simulink model "szalwach_mroz_perlinski"  (R2015a)
settings: Solver=ode45  StartTime=0.0  StopTime=200  RelTol=1e-3
settings Model: Creator=bszal  LastModifiedBy=bszal

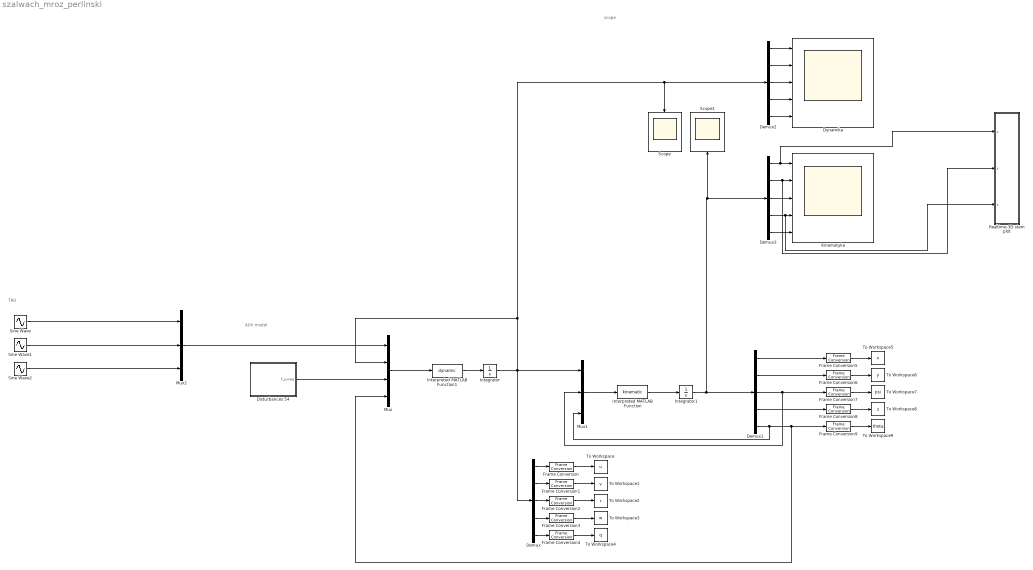
== system szalwach_mroz_perlinski ==
  note: scope
  note: TAU
  note: AUV model
  Demux{,1..3} (4 alike) : Demux  Outputs=5
  Disturbances 54 : Subsystem
  "Dynamika " : Scope  NumInputPorts=5
      settings: YMin=-5~-5~-5~-5~-5  YMax=5~5~5~5~5
  Frame Conversion{,1..9} (10 alike) : FrameConversion  OutFrame=Sample-based
  Integrator : Integrator  InitialCondition=[0;0;0;0;0]
  Integrator1 : Integrator  InitialCondition=[0;0;0;0;0]
  Interpreted MATLAB Function : MATLABFcn  MATLABFcn=kinematic  OutputDimensions=5
  Interpreted MATLAB Function1 : MATLABFcn  MATLABFcn=dynamic  OutputDimensions=5
  Kinematyka : Scope  NumInputPorts=5
      settings: YMin=-5~-5~-5~-5~-5  YMax=5~5~5~5~5  SaveName=ScopeData2
  Mux : Mux
  Mux1 : Mux  Inputs=3
  Mux2 : Mux  Inputs=3
  Realtime-3D stem plot : MATLAB Function  TreatAsAtomicUnit=on
  Scope : Scope
      settings: SaveName=ScopeData3
  Scope1 : Scope
      settings: SaveName=ScopeData4
  Sine Wave : Sin  SampleTime=0
  Sine Wave1 : Sin  SampleTime=0
  Sine Wave2 : Sin  SampleTime=0
  To Workspace : ToWorkspace  VariableName=u  SaveFormat=Timeseries  SampleTime=-1
  To Workspace1 : ToWorkspace  VariableName=v  SaveFormat=Timeseries  SampleTime=-1
  To Workspace2 : ToWorkspace  VariableName=r  SaveFormat=Timeseries  SampleTime=-1
  To Workspace3 : ToWorkspace  VariableName=w  SaveFormat=Timeseries  SampleTime=-1
  To Workspace4 : ToWorkspace  VariableName=q  SaveFormat=Timeseries  SampleTime=-1
  To Workspace5 : ToWorkspace  VariableName=x  SaveFormat=Timeseries  SampleTime=-1
  To Workspace6 : ToWorkspace  VariableName=y  SaveFormat=Timeseries  SampleTime=-1
  To Workspace7 : ToWorkspace  VariableName=psi  SaveFormat=Timeseries  SampleTime=-1
  To Workspace8 : ToWorkspace  VariableName=z  SaveFormat=Timeseries  SampleTime=-1
  To Workspace9 : ToWorkspace  VariableName=theta  SaveFormat=Timeseries  SampleTime=-1
  wires:
  Mux2/1 -> Mux/1
  Disturbances 54/1(f_uvrwq) -> Mux/3
  Interpreted MATLAB Function1/1 -> Integrator/1
  Mux/1 -> Interpreted MATLAB Function1/1
  Integrator/1 -> Scope/1, Demux2/1, Mux/2, Demux/1, Mux1/1
  Demux/1 -> Frame Conversion/1
  Demux/2 -> Frame Conversion1/1
  Demux/3 -> Frame Conversion2/1
  Frame Conversion/1 -> To Workspace/1
  Frame Conversion1/1 -> To Workspace1/1
  Frame Conversion2/1 -> To Workspace2/1
  Frame Conversion3/1 -> To Workspace3/1
  Demux/4 -> Frame Conversion3/1
  Demux/5 -> Frame Conversion4/1
  Frame Conversion4/1 -> To Workspace4/1
  Mux1/1 -> Interpreted MATLAB Function/1
  Interpreted MATLAB Function/1 -> Integrator1/1
  Integrator1/1 -> Demux1/1, Demux3/1, Scope1/1
  Demux1/1 -> Frame Conversion5/1
  Demux1/2 -> Frame Conversion6/1
  Demux1/3 -> Mux1/2, Frame Conversion7/1
  Frame Conversion5/1 -> To Workspace5/1
  Frame Conversion6/1 -> To Workspace6/1
  Frame Conversion7/1 -> To Workspace7/1
  Frame Conversion8/1 -> To Workspace8/1
  Demux1/4 -> Frame Conversion8/1
  Demux1/5 -> Mux1/3, Mux/4, Frame Conversion9/1
  Frame Conversion9/1 -> To Workspace9/1
  Demux2/1 -> "Dynamika "/1
  Demux2/2 -> "Dynamika "/2
  Demux2/3 -> "Dynamika "/3
  Demux2/4 -> "Dynamika "/4
  Demux2/5 -> "Dynamika "/5
  Demux3/1 -> Realtime-3D stem plot/1(x), Kinematyka/1
  Demux3/2 -> Realtime-3D stem plot/2(y), Kinematyka/2
  Demux3/3 -> Kinematyka/3
  Demux3/4 -> Realtime-3D stem plot/3(z), Kinematyka/4
  Demux3/5 -> Kinematyka/5
  Sine Wave/1 -> Mux2/1
  Sine Wave1/1 -> Mux2/2
  Sine Wave2/1 -> Mux2/3

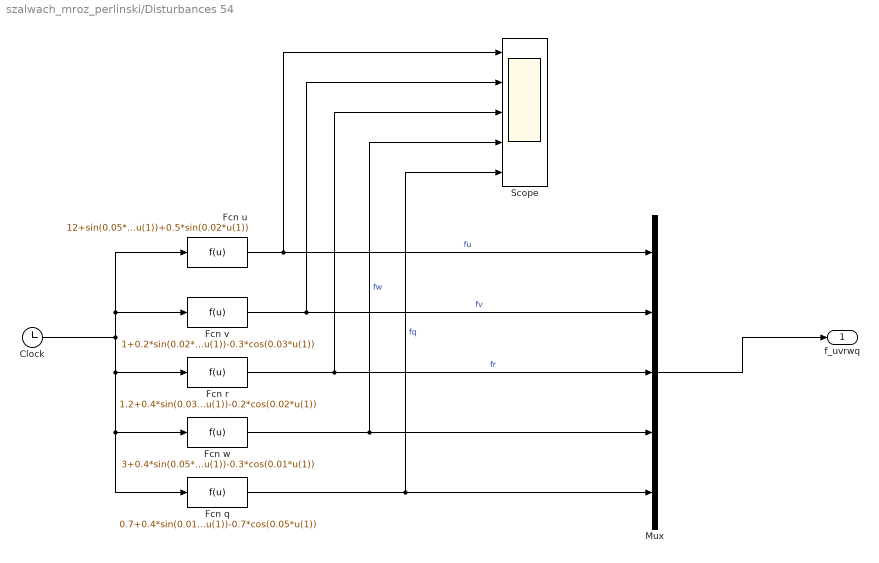
== system szalwach_mroz_perlinski/Disturbances 54 ==
  Clock : Clock
  Fcn q : Fcn  Expr=0.7+0.4*sin(0.01*u(1))-0.7*cos(0.05*u(1))
  Fcn r : Fcn  Expr=1.2+0.4*sin(0.03*u(1))-0.2*cos(0.02*u(1))
  Fcn u : Fcn  Expr=12+sin(0.05*u(1))+0.5*sin(0.02*u(1))
  Fcn v : Fcn  Expr=1+0.2*sin(0.02*u(1))-0.3*cos(0.03*u(1))
  Fcn w : Fcn  Expr=3+0.4*sin(0.05*u(1))-0.3*cos(0.01*u(1))
  Mux : Mux  Inputs=5
  Scope : Scope  NumInputPorts=5
      settings: YMin=-5~-5~-5~-5~-5  YMax=5~5~5~5~5
  f_uvrwq : Outport
  wires:
  Clock/1 -> Fcn v/1, Fcn u/1, Fcn q/1, Fcn w/1, Fcn r/1
  Fcn v/1 -> Scope/2, Mux/2  "fv"
  Fcn u/1 -> Scope/1, Mux/1  "fu"
  Fcn r/1 -> Scope/3, Mux/3  "fr"
  Fcn w/1 -> Scope/4, Mux/4  "fw"
  Fcn q/1 -> Scope/5, Mux/5  "fq"
  Mux/1 -> f_uvrwq/1

== matlab function szalwach_mroz_perlinski/Realtime-3D stem plot ==
  data: x input; y input; z input
function  fcn(x, y, z)
figure(1);
hold on; grid on;
coder.extrinsic('stem3');
stem3(x, y, z, 'd', 'k' );

% coder.extrinsic('plot3');
% plot3(x, y, z, 'd', 'k' );
% plot3(x1, y1, z1, '+', 'm' );

view([45 45]);
